simulink model "final_model"  (R2024b)
settings: Solver=ode4  StartTime=0.0  StopTime=4/50  RelTol=1e-3
libraries: spsIGBTLib x6, spsThyristorLib x4, spsVoltageMeasurementLib x4, spsParallelRLCBranchLib x3, spsSeriesRLCBranchLib x2, spsACVoltageSourceLib x1, spsAsynchronousMachineSIUnitsLib x1, spsGroundLib x1, spsThreePhaseVIMeasurementLib x1, spsTriangleGeneratorLib x1, sps_lib x1
settings Model: Creator=Abhijith_Kumble  LastModifiedBy=Abhijith_Kumble

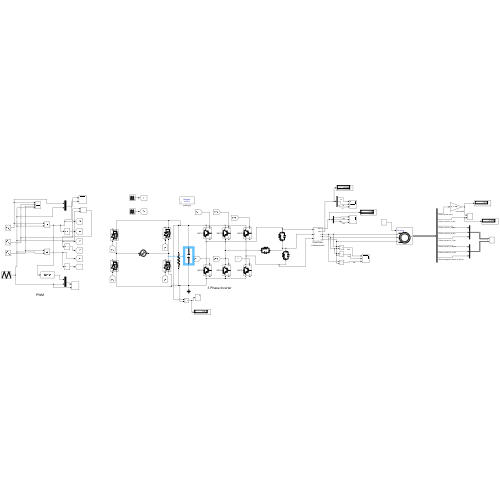
[thumbnail: Simulink's stored preview of the top-level diagram]
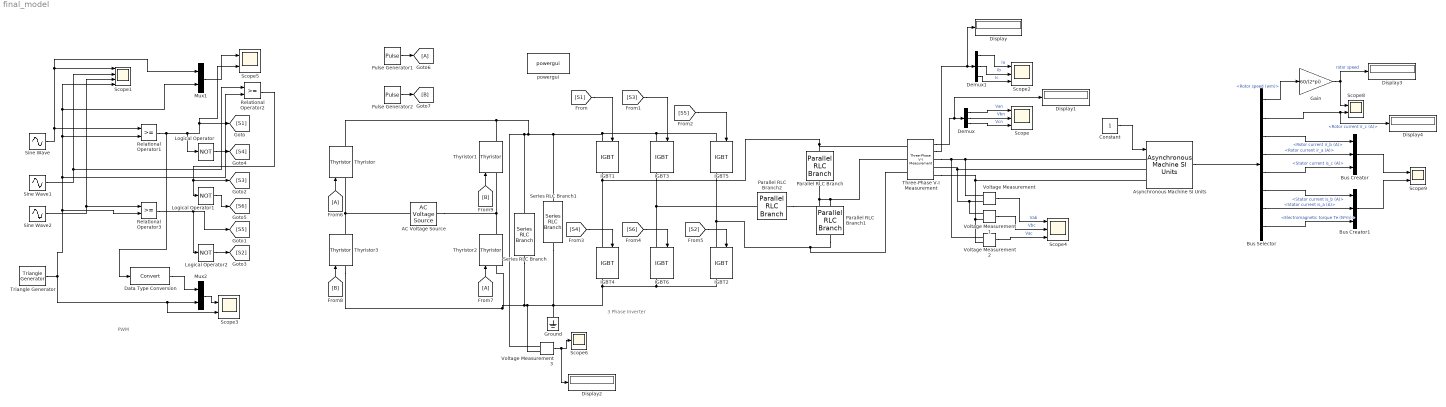
== system final_model ==
  note: PWM
  note: 3 Phase Inverter
  AC Voltage Source : spsACVoltageSourceLib/AC Voltage Source  Amplitude=700  Phase=0  Frequency=50  SampleTime=0  Measurements=None  BusType=swing  Pref=10e3  Qref=0  Qmin=-inf  Qmax=+inf
  Asynchronous Machine SI Units : spsAsynchronousMachineSIUnitsLib/Asynchronous Machine SI Units  RotorType=Squirrel-cage  PresetModel="15:  5.4 HP (4KW)   400 V  50Hz 1430 RPM"  MechanicalLoad=Torque Tm  ShowDetailedParameters=on  ReferenceFrame=Rotor  Units=SI  MeasurementBus=off  NominalParameters=[4000 400 50]  VoltageRatio=1  Stator=[1.405 0.005839]  Rotor=[1.395 0.005839]  Cage1=[0.4155 0.002066]  Cage2=[0.4168 0.0003495]  Lm=0.1722  Mechanical=[0.0131 0.002985 2]  PolePairs=2  InitialConditions=[0 0 0 0 0 0 0 0]  SimulateSaturation=off  Saturation=[14.03593122, 27.81365428, 53.79336849, 72.68890987, 97.98006896, 148.6815601, 215.7428561, 302.9841135, 428.7778367 ; 230, 322, 414, 460, 506, 552, 598, 644, 690]  LoadFlowParameters=1492000  TsPowergui=0  TsBlock=-1  IterativeModel=Trapezoidal non iterative  IterativeDiscreteModel=Trapezoidal non iterative  Pmec=1.492e+006
  Bus Creator : BusCreator  Inputs=3
  Bus Creator1 : BusCreator  Inputs=3
  Bus Selector : BusSelector  OutputSignals=Mechanical.Rotor speed (wm),Rotor measurements.Rotor current ir_c (A),Rotor measurements.Rotor current ir_b (A),Rotor measurements.Rotor current ir_a (A),Stator measurements.Stator current is_c (A),Stator measurements.Stator current is_b (A),Stator measurements.Stator current is_a (A),Mechanical.Electromagnetic torque Te (N*m)
  Constant : Constant
  Data Type Conversion : DataTypeConversion  SaturateOnIntegerOverflow=off  RndMeth=Floor
  Demux : Demux  Outputs=3
  Demux1 : Demux  Outputs=3
  Display{,1..4} (5 alike) : Display
  From6 : From
  From7 : From
  Gain : Gain  Gain=60/(2*pi)
  Goto6 : Goto
  Ground : spsGroundLib/Ground  LConnTagsString=a
  IGBT{1..6} (6 alike) : spsIGBTLib/IGBT  Ron=0.001  Lon=0  Vf=1  Tf=1e-6  Tt=2e-6  IC=0  Rs=1e5  Cs=inf  Measurements=on
  Logical Operator : Logic  Operator=NOT  AllPortsSameDT=off  OutDataTypeStr=boolean
  Logical Operator1 : Logic  Operator=NOT  AllPortsSameDT=off  OutDataTypeStr=boolean
  Logical Operator2 : Logic  Operator=NOT  AllPortsSameDT=off  OutDataTypeStr=boolean
  Mux1 : Mux  Inputs=2
  Mux2 : Mux  Inputs=2
  Parallel RLC Branch : spsParallelRLCBranchLib/Parallel RLC Branch  LConnTagsString=a  RConnTagsString=__new0  BranchType=RC  Resistance=10  Inductance=1e-3  SetiL0=off  InitialCurrent=0  Capacitance=100  Setx0=off  InitialVoltage=0  Measurements=None
  Parallel RLC Branch1 : spsParallelRLCBranchLib/Parallel RLC Branch  LConnTagsString=a  RConnTagsString=__new0  BranchType=RC  Resistance=10  Inductance=1e-3  SetiL0=off  InitialCurrent=0  Capacitance=100  Setx0=off  InitialVoltage=0  Measurements=None
  Parallel RLC Branch2 : spsParallelRLCBranchLib/Parallel RLC Branch  LConnTagsString=a  RConnTagsString=__new0  BranchType=RC  Resistance=10  Inductance=1e-3  SetiL0=off  InitialCurrent=0  Capacitance=100  Setx0=off  InitialVoltage=0  Measurements=None
  Pulse Generator1 : DiscretePulseGenerator  PulseType=Time based  Period=0.02  PulseWidth=5  PhaseDelay=0.0033
  Pulse Generator2 : DiscretePulseGenerator  PulseType=Time based  Period=0.02  PulseWidth=5  PhaseDelay=0.0133
  Relational Operator1 : RelationalOperator  OutDataTypeStr=boolean  InputSameDT=off
  Relational Operator2 : RelationalOperator  OutDataTypeStr=boolean  InputSameDT=off
  Relational Operator3 : RelationalOperator  OutDataTypeStr=boolean  InputSameDT=off
  Scope : Scope  NumInputPorts=3
  Scope1 : Scope  NumInputPorts=4
  Scope2 : Scope  NumInputPorts=3
  Scope{3,5,8..9} (4 alike) : Scope  NumInputPorts=2
  Scope4 : Scope  NumInputPorts=3
  Scope6 : Scope
  Series RLC Branch : spsSeriesRLCBranchLib/Series RLC Branch  LConnTagsString=__new0  RConnTagsString=__new0  BranchType=R  Resistance=10  Inductance=1e-3  SetiL0=off  InitialCurrent=0  Capacitance=1e-6  Setx0=off  InitialVoltage=0  Measurements=None
  Series RLC Branch1 : spsSeriesRLCBranchLib/Series RLC Branch  LConnTagsString=__new0  RConnTagsString=__new0  BranchType=C  Resistance=1  Inductance=1e-3  SetiL0=off  InitialCurrent=0  Capacitance=100  Setx0=off  InitialVoltage=0  Measurements=None
  Sine Wave : Sin  Frequency=2*pi*50  SampleTime=0
  Sine Wave1 : Sin  Frequency=2*pi*50  Phase=2*pi/3  SampleTime=0
  Sine Wave2 : Sin  Frequency=2*pi*50  Phase=-2*pi/3  SampleTime=0
  Three-Phase V-I Measurement : spsThreePhaseVIMeasurementLib/Three-Phase V-I Measurement  VoltageMeasurement=phase-to-phase  SetLabelV=off  LabelV=Vabc  Vpu=off  VpuLL=off  CurrentMeasurement=yes  SetLabelI=off  LabelI=Iabc  Ipu=off  Pbase=100e6  Vbase=500e3  OutputType=Complex  PhasorSimulation=off  PSBequivalent=0
  Thyristor{,1..3} (4 alike) : spsThyristorLib/Thyristor  Ron=0.001  Lon=0  Vf=0.8  IC=0  Rs=500  Cs=250e-9  Measurements=on
  Triangle Generator : spsTriangleGeneratorLib/Triangle Generator  Freq=25e3  Phase=0  Ts=0
  Voltage Measurement{,1..3} (4 alike) : spsVoltageMeasurementLib/Voltage Measurement  PhasorSimulation=off  OutputType=Complex  PSBequivalent=0
  powergui : sps_lib/powergui  Priority=1  SimulationMode=Discrete  SampleTime=10e-6  frequency=60  Iterations=50  frequencyindice=0  Pbase=100e6  ErrMax=1e-4  UnitsV=kV  UnitsW=MW  buscounter=0  FunctionMessages=off  echomessages=off  EnableUseOfTLC=off  CurrentSourceSwitches=off  DisableSnubberDevices=off  DisableRonSwitches=off  DisableVfSwitches=off  DisplayEquations=off  AutomaticDiscreteSolvers=off  SolverType=Tustin/Backward Euler (TBE)  Interpol=off  ExternalGateDelay=off  methode=off  Ts=100  x0status=blocks  SPID=on  SwTol=0  HookPort=off  NonlinearTolerance=1e-4  nMaxIteration=100  ContinueOnMaxIteration=off  RestoreLinks=warning  ResistiveCurrentMeasurement=off  Frange=[0:2:500]  Ylog=off  Xlog=on  ShowGrid=off  save=off  variable=ZData  structure=0  ZoomFFT=off  StartTime=0.0  cycles=1  DisplayStyle=1  fundamental=60  FreqAxis=off  MaxFrequency=1000  frequencyindicesteady=1  RmsSteady=1  display=off
  wires:
  Relational Operator1/1 -> Data Type Conversion/1, Scope5/2, [S1], Logical Operator/1
  Demux/3 -> Scope/3  "Vcn"
  Demux/1 -> Scope/1  "Van"
  [S1] -> IGBT1/1
  [S2] -> IGBT2/1
  Voltage Measurement2/1 -> Scope4/3  "Vac"
  Sine Wave1/1 -> Scope1/2, Relational Operator2/1
  Mux2/1 -> Scope3/1
  [S6] -> IGBT6/1
  Relational Operator2/1 -> [S3], Logical Operator1/1
  Logical Operator1/1 -> [S6]
  Sine Wave/1 -> Scope1/1, Mux1/1, Relational Operator1/1
  [S4] -> IGBT4/1
  Logical Operator2/1 -> [S2]
  Three-Phase V-I Measurement/1 -> Display1/1, Demux/1
  Demux1/2 -> Scope2/2  "Ib"
  Relational Operator3/1 -> [S5], Logical Operator2/1
  [S3] -> IGBT3/1
  Demux/2 -> Scope/2  "Vbn"
  Sine Wave2/1 -> Scope1/3, Relational Operator3/1
  Triangle Generator/1 -> Scope3/2, Mux2/2, Scope1/4, Mux1/2, Relational Operator1/2, Relational Operator2/2, Relational Operator3/2
  Voltage Measurement1/1 -> Scope4/2  "Vbc"
  Demux1/3 -> Scope2/3  "Ic"
  Demux1/1 -> Scope2/1  "Ia"
  Voltage Measurement/1 -> Scope4/1  "Vab"
  Data Type Conversion/1 -> Mux2/1
  Mux1/1 -> Scope5/1
  [S5] -> IGBT5/1
  Three-Phase V-I Measurement/2 -> Display/1, Demux1/1
  Logical Operator/1 -> [S4]
  Pulse Generator1/1 -> Goto6/1
  From7/1 -> Thyristor2/1
  [B] -> Thyristor3/1
  Pulse Generator2/1 -> [B]
  From6/1 -> Thyristor/1
  [B] -> Thyristor1/1
  Voltage Measurement3/1 -> Display2/1, Scope6/1
  Bus Selector/1 -> Gain/1  "<Rotor speed (wm)>"
  Bus Selector/5 -> Bus Creator/3  "<Stator current is_c (A)>"
  Bus Selector/6 -> Bus Creator1/1  "<Stator current is_b (A)>"
  Asynchronous Machine SI Units/1 -> Bus Selector/1
  Gain/1 -> Scope8/1, Display3/1  "rotor speed"
  Bus Creator/1 -> Scope9/1
  Bus Selector/7 -> Bus Creator1/2  "<Stator current is_a (A)>"
  Bus Selector/3 -> Bus Creator/1  "<Rotor current ir_b (A)>"
  Bus Creator1/1 -> Scope9/2
  Bus Selector/2 -> Display4/1, Scope8/2  "<Rotor current ir_c (A)>"
  Constant/1 -> Asynchronous Machine SI Units/1
  Bus Selector/8 -> Bus Creator1/3  "<Electromagnetic torque Te (N*m)>"
  Bus Selector/4 -> Bus Creator/2  "<Rotor current ir_a (A)>"
  connections:
  Parallel RLC Branch2/LConn1 -- Parallel RLC Branch1/LConn1 -- Three-Phase V-I Measurement/LConn2 -- Parallel RLC Branch/RConn1
  Three-Phase V-I Measurement/RConn3 -- Asynchronous Machine SI Units/LConn3 -- Voltage Measurement2/LConn2 -- Voltage Measurement1/LConn2
  Thyristor3/LConn1 -- Series RLC Branch/RConn1 -- IGBT4/RConn1 -- IGBT2/RConn1 -- IGBT6/RConn1 -- Series RLC Branch1/RConn1 -- Ground/LConn1 -- Voltage Measurement3/LConn2 -- Thyristor2/LConn1
  IGBT5/RConn1 -- Three-Phase V-I Measurement/LConn3 -- Parallel RLC Branch1/RConn1 -- IGBT2/LConn1
  Voltage Measurement/LConn2 -- Voltage Measurement1/LConn1 -- Three-Phase V-I Measurement/RConn2 -- Asynchronous Machine SI Units/LConn2
  IGBT1/RConn1 -- IGBT4/LConn1 -- Three-Phase V-I Measurement/LConn1 -- Parallel RLC Branch/LConn1
  AC Voltage Source/RConn1 -- Thyristor3/RConn1 -- Thyristor/LConn1
  Thyristor1/LConn1 -- AC Voltage Source/LConn1 -- Thyristor2/RConn1
  IGBT5/LConn1 -- IGBT3/LConn1 -- Voltage Measurement3/LConn1 -- Series RLC Branch/LConn1 -- Thyristor/RConn1 -- Thyristor1/RConn1 -- Series RLC Branch1/LConn1 -- IGBT1/LConn1
  IGBT3/RConn1 -- Parallel RLC Branch2/RConn1 -- IGBT6/LConn1
  Three-Phase V-I Measurement/RConn1 -- Voltage Measurement2/LConn1 -- Voltage Measurement/LConn1 -- Asynchronous Machine SI Units/LConn1
